simulink model "test_mux_euler"  (Simulink 7.6)
settings: Solver=ode45  StartTime=0.0  StopTime=10.0  RelTol=1e-3
libraries: simulink x4
settings Model: Creator=jporter  LastModifiedBy=jporter

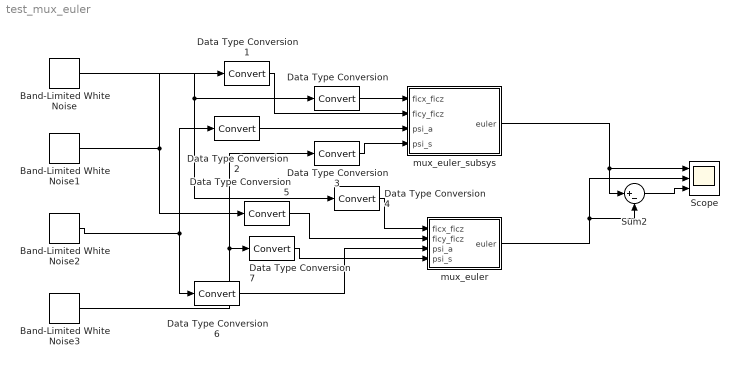
== system test_mux_euler ==
  Band-Limited White Noise{,1..3} (4 alike) : simulink/Sources/Band-Limited White Noise  SystemSampleTime=-1  Cov=0.5  Ts=0.01  seed=[23341]
  Data Type Conversion{,1..7} (8 alike) : DataTypeConversion
  Scope : Scope  NumInputPorts=3
      settings: YMin=-5~-5~-5  YMax=5~5~5
  Sum2 : Sum  Inputs=|+-
  mux_euler : Stateflow chart  TreatAsAtomicUnit=on
  mux_euler_subsys : Subsystem
  wires:
  Band-Limited White Noise/1 -> Data Type Conversion/1, Data Type Conversion4/1
  Band-Limited White Noise1/1 -> Data Type Conversion1/1, Data Type Conversion5/1
  Band-Limited White Noise2/1 -> Data Type Conversion2/1, Data Type Conversion6/1
  Band-Limited White Noise3/1 -> Data Type Conversion3/1, Data Type Conversion7/1
  Data Type Conversion/1 -> mux_euler_subsys/1(ficx_ficz)
  Data Type Conversion1/1 -> mux_euler_subsys/2(ficy_ficz)
  Data Type Conversion2/1 -> mux_euler_subsys/3(psi_a)
  Data Type Conversion3/1 -> mux_euler_subsys/4(psi_s)
  Data Type Conversion4/1 -> mux_euler/1(ficx_ficz)
  Data Type Conversion5/1 -> mux_euler/2(ficy_ficz)
  Data Type Conversion6/1 -> mux_euler/3(psi_a)
  Data Type Conversion7/1 -> mux_euler/4(psi_s)
  mux_euler_subsys/1(euler) -> Scope/1, Sum2/1
  Sum2/1 -> Scope/3
  mux_euler/1(euler) -> Scope/2, Sum2/2

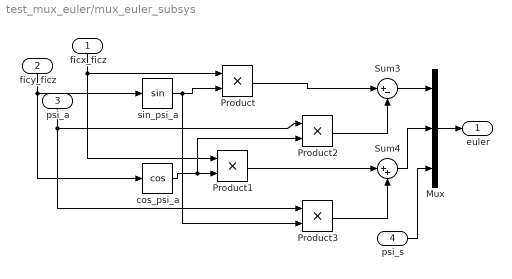
== system test_mux_euler/mux_euler_subsys ==
  ficx_ficz : Inport
  ficy_ficz : Inport  Port=2
  psi_a : Inport  Port=3
  psi_s : Inport  Port=4
  Mux : Mux  Inputs=3
  Product{,1..3} (4 alike) : Product  RndMeth=Zero
  Sum3 : Sum  Inputs=|+-
  Sum4 : Sum  Inputs=|++
  cos_psi_a : Trigonometry  Operator=cos
  sin_psi_a : Trigonometry
  euler : Outport
  wires:
  sin_psi_a/1 -> Product/2, Product3/2
  Product/1 -> Sum3/1
  cos_psi_a/1 -> Product2/2, Product1/2
  Product2/1 -> Sum3/2
  Product1/1 -> Sum4/1
  Product3/1 -> Sum4/2
  Sum3/1 -> Mux/1
  Sum4/1 -> Mux/2
  ficx_ficz/1 -> Product/1, Product1/1
  ficy_ficz/1 -> sin_psi_a/1, cos_psi_a/1
  psi_a/1 -> Product2/1, Product3/1
  Mux/1 -> euler/1
  psi_s/1 -> Mux/3

== matlab function mux_euler ==
  data: ficx_ficz input single size=[1]; euler output single size=[3]; ficy_ficz input single size=[1]; psi_a input single size=[1]; psi_s input single size=[1]
function euler = fcn(ficx_ficz, ficy_ficz, psi_a, psi_s)
% This block supports the Embedded MATLAB subset.
% See the help menu for details. 

A = [sin(psi_a) -cos(psi_a); cos(psi_a) sin(psi_a)];
% Get [phi, theta] 
euler_angs = (A * [ficx_ficz; ficy_ficz])';

euler=[euler_angs(1);euler_angs(2);psi_s];
